simulink model "pid"  (Simulink 7.3)
settings: Solver=ode45  StartTime=0.0  StopTime=1200  RelTol=1e-3
settings Model: Creator=Administrator  LastModifiedBy=sn00632
settings DataIOCC: LimitDataPoints=off
settings OptimizationCC: InlineInvariantSignals=on  InitFltsAndDblsToZero=on
settings DebuggingCC: SaveWithParameterizedLinksMsg=none  SignalResolutionControl=TryResolveAllWithWarning  SolverPrmCheckMsg=none  MultiTaskDSMMsg=warning  MultiTaskCondExecSysMsg=none  StrictBusMsg=None
settings RTWCC: IncludeERTFirstTime=on
settings GRTTargetCC: TargetFcnLib=ansi_tfl_tmw.mat

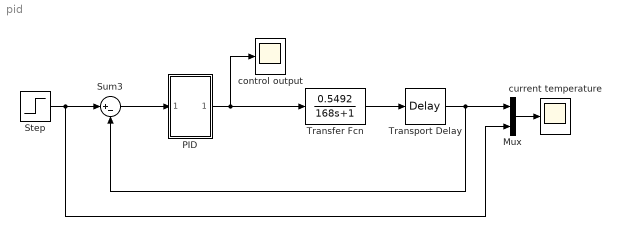
== system pid ==
  Mux : Mux  Inputs=2
  PID : Subsystem  mask(PID parameters){P=2.8, I=0.0156, D=12}
      mask prompts: P "Proportion coefficient"; I "Integral coefficient"; D "Differential coefficient"
      mask help: Adjust PID control parameters
      mask Display: image(imread('tubiao.jpg'))
  Step : Step  Time=0  After=80  SampleTime=0
  Sum3 : Sum  Inputs=|+-  OutDataType=sfix(16)  OutScaling=2^0
  Transfer Fcn : TransferFcn  Numerator=[0.5492]  Denominator=[168 1]
  Transport Delay : TransportDelay  DelayTime=58.5
  control output : Scope
      settings: TimeRange=1200  YMin=-20  YMax=500
  current temperature : Scope
      settings: TimeRange=2.920617309618137  YMin=61.3913  YMax=61.649
  wires:
  Transport Delay/1 -> Sum3/2, Mux/1
  PID/1(Out1) -> Transfer Fcn/1, control output/1
  Step/1 -> Sum3/1, Mux/2
  Transfer Fcn/1 -> Transport Delay/1
  Mux/1 -> current temperature/1
  Sum3/1 -> PID/1(In1)

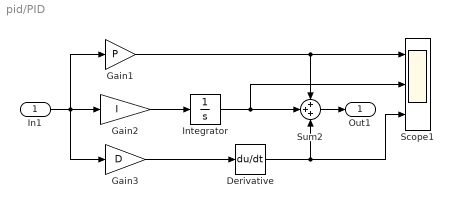
== system pid/PID ==
  In1 : Inport
  Derivative : Derivative
  Gain1 : Gain  Gain=P  ParameterDataType=sfix(16)  ParameterScaling=2^0  OutDataType=sfix(16)  OutScaling=2^0
  Gain2 : Gain  Gain=I  ParameterDataType=sfix(16)  ParameterScaling=2^0  OutDataType=sfix(16)  OutScaling=2^0
  Gain3 : Gain  Gain=D  ParameterDataType=sfix(16)  ParameterScaling=2^0  OutDataType=sfix(16)  OutScaling=2^0
  Integrator : Integrator
  Scope1 : Scope  NumInputPorts=3
      settings: TimeRange=1200  YMin=0~-5~-15  YMax=20~5~5
  Sum2 : Sum  Inputs=+++  OutDataType=sfix(16)  OutScaling=2^0
  Out1 : Outport
  wires:
  Gain1/1 -> Sum2/1, Scope1/1
  Derivative/1 -> Sum2/3, Scope1/3
  Integrator/1 -> Sum2/2, Scope1/2
  Gain2/1 -> Integrator/1
  Gain3/1 -> Derivative/1
  In1/1 -> Gain1/1, Gain3/1, Gain2/1
  Sum2/1 -> Out1/1
